simulink model "IFCC_SIMULATION"  (R2018a)
settings: Solver=VariableStepAuto  StartTime=0.0  StopTime=10.0  RelTol=1e-3
libraries: simulink x25
(part 1 of 2)
settings Model: Creator=vsbdh  LastModifiedBy=vsbdh

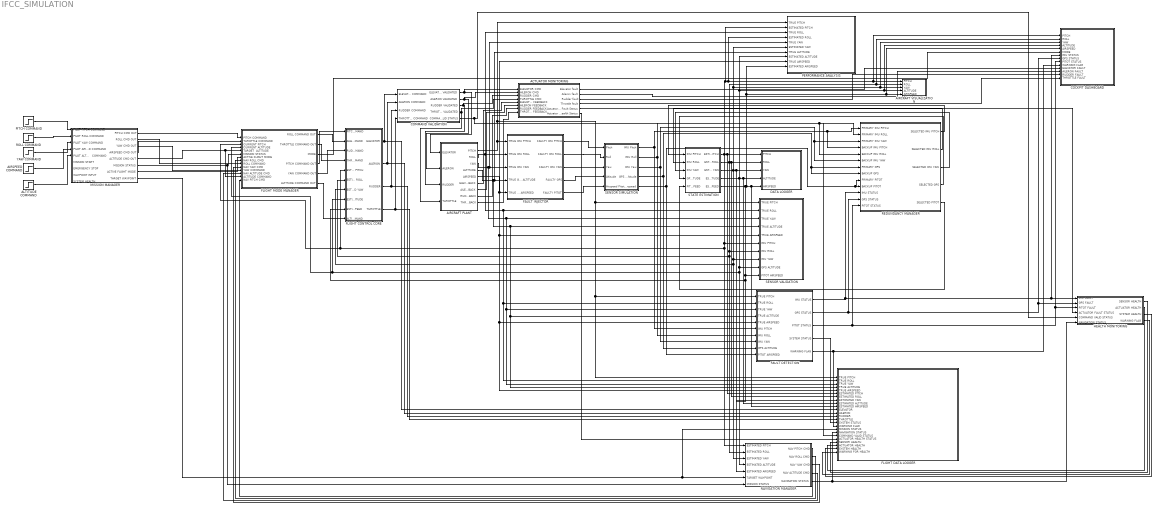
== system IFCC_SIMULATION ==
  " MISSION MANAGER" : Subsystem
  " SENSOR VALIDATION" : Subsystem
  ACTUATOR MONITORING : Subsystem
  AIRCRAFT PLANT : Subsystem
  AIRCRAFT VISUALIZATION : Subsystem
  AIRSPEED COMMAND : Step  Time=0  SampleTime=0
  ALTITUDE COMMAND : Step  Time=2  After=1000  SampleTime=0
  COCKPIT DASHBOARD : Subsystem
  COMMAND VALIDATION : Subsystem
  DATA LOGGER : Subsystem
  FAULT DETECTION : Subsystem
  "FAULT INJECTOR " : Subsystem
  FLIGHT CONTROL CORE : Subsystem
  FLIGHT DATA LOGGER : Subsystem
  FLIGHT MODE MANAGER : Subsystem
  HEALTH MONITORING : Subsystem
  NAVIGATION MANAGER : Subsystem
  PERFORMANCE ANALYSIS : Subsystem
  PITCH COMMAND : Step  Time=0  SampleTime=0
  REDUNDANCY MANAGER : Subsystem
  ROLL COMMAND : Step  Time=0  SampleTime=0
  SENSOR SIMULATION : Subsystem
  STATE ESTIMATION : Subsystem
  YAW COMMAND : Step  Time=0  SampleTime=0
  wires:
  SENSOR SIMULATION/2(IMU Roll) -> REDUNDANCY MANAGER/2(PRIMARY IMU ROLL), REDUNDANCY MANAGER/5(BACKUP IMU ROLL), FAULT DETECTION/7(IMU ROLL)
  FLIGHT CONTROL CORE/4(THROTTLE) -> COMMAND VALIDATION/4(THROTTLE COMMAND), FLIGHT DATA LOGGER/14(THROTTLE)
  REDUNDANCY MANAGER/2(SELECTED IMU ROLL) -> STATE ESTIMATION/2(IMU ROLL)
  "FAULT INJECTOR "/5(FAULTY PITOT) -> SENSOR SIMULATION/5(Airspeed)
  FLIGHT MODE MANAGER/3(MODE) -> COCKPIT DASHBOARD/6(MODE)
  FLIGHT CONTROL CORE/3(RUDDER) -> FLIGHT DATA LOGGER/13(RUDDER), COMMAND VALIDATION/3(RUDDER COMMAND)
  FAULT DETECTION/1(IMU STATUS) -> HEALTH MONITORING/1(IMU FAULT), COCKPIT DASHBOARD/7(IMU STATUS), REDUNDANCY MANAGER/11(IMU STATUS)
  ALTITUDE COMMAND/1 -> " MISSION MANAGER"/5(PILOT ALTITUDE   COMMAND)
  "FAULT INJECTOR "/2(FAULTY IMU ROLL) -> SENSOR SIMULATION/2(Roll)
  "FAULT INJECTOR "/1(FAULTY IMU PITCH) -> SENSOR SIMULATION/1(Pitch)
  "FAULT INJECTOR "/3(FAULTY IMU YAW) -> SENSOR SIMULATION/3(Yaw)
  FAULT DETECTION/5(WARNING FLAG) -> FLIGHT DATA LOGGER/16(WARNING FLAG), COCKPIT DASHBOARD/10(WARNING FLAG)
  REDUNDANCY MANAGER/5(SELECTED PITOT) -> STATE ESTIMATION/5(PITOT AIRSPEED)
  REDUNDANCY MANAGER/3(SELECTED IMU YAW) -> STATE ESTIMATION/3(IMU YAW)
  REDUNDANCY MANAGER/1(SELECTED IMU PITCH) -> STATE ESTIMATION/1(IMU PITCH)
  REDUNDANCY MANAGER/4(SELECTED GPS) -> STATE ESTIMATION/4(GPS ALTITUDE)
  FAULT DETECTION/2(GPS STATUS) -> HEALTH MONITORING/2(GPS FAULT), COCKPIT DASHBOARD/8(GPS STATUS), REDUNDANCY MANAGER/12(GPS STATUS)
  FAULT DETECTION/3(PITOT STATUS) -> HEALTH MONITORING/3(PITOT FAULT), COCKPIT DASHBOARD/9(PITOT STATUS), REDUNDANCY MANAGER/13(PITOT STATUS)
  FAULT DETECTION/4(SYSTEM STATUS) -> FLIGHT DATA LOGGER/15(SYSTEM STATUS)
  YAW COMMAND/1 -> " MISSION MANAGER"/3(PILOT YAW COMMAND)
  FLIGHT MODE MANAGER/1(ROLL COMMAND OUT) -> FLIGHT CONTROL CORE/2(AILERON COMMAND)
  PITCH COMMAND/1 -> " MISSION MANAGER"/1(PILOT PITCH COMMAND)
  FLIGHT CONTROL CORE/1(ELEVATOR) -> COMMAND VALIDATION/1(ELEVATOR COMMAND), FLIGHT DATA LOGGER/11(ELEVATOR)
  FLIGHT MODE MANAGER/2(THROTTLE COMMAND OUT) -> FLIGHT CONTROL CORE/4(THROTTLE COMMAND)
  ROLL COMMAND/1 -> " MISSION MANAGER"/2(PILOT ROLL COMMAND)
  SENSOR SIMULATION/4(GPS Altitude) -> FAULT DETECTION/9(GPS ALTITUDE), REDUNDANCY MANAGER/8(BACKUP GPS), REDUNDANCY MANAGER/7(PRIMARY GPS)
  STATE ESTIMATION/2(ESTIMATED ROLL) -> NAVIGATION MANAGER/2(ESTIMATED ROLL), FLIGHT CONTROL CORE/6(ESTIMATED ROLL), " SENSOR VALIDATION"/7(IMU ROLL), COCKPIT DASHBOARD/2(ROLL), AIRCRAFT VISUALIZATION/2(ROLL), FLIGHT DATA LOGGER/7(ESTIMATED ROLL), DATA LOGGER/2(ROLL)
  AIRSPEED COMMAND/1 -> " MISSION MANAGER"/4(PILOT AIRSPEED COMMAND)
  STATE ESTIMATION/3(ESTIMATED YAW) -> NAVIGATION MANAGER/3(ESTIMATED YAW), FLIGHT CONTROL CORE/7(ESTIMATED YAW), " SENSOR VALIDATION"/8(IMU YAW), PERFORMANCE ANALYSIS/6(ESTIMATED YAW), COCKPIT DASHBOARD/3(YAW), AIRCRAFT VISUALIZATION/3(YAW), FLIGHT DATA LOGGER/8(ESTIMATED YAW), DATA LOGGER/3(YAW)
  STATE ESTIMATION/5(ESTIMATED AIRSPEED) -> PERFORMANCE ANALYSIS/10(ESTIMATED AIRSPEED), COCKPIT DASHBOARD/5(AIRSPEED), AIRCRAFT VISUALIZATION/5(AIRSPEED), FLIGHT DATA LOGGER/10(ESTIMATED AIRSPEED), DATA LOGGER/5(AIRSPEED), NAVIGATION MANAGER/5(ESTIMATED AIRSPEED), FLIGHT CONTROL CORE/9(ESTIMATED AIRSPEED), " SENSOR VALIDATION"/10(PITOT AIRSPEED)
  STATE ESTIMATION/1(ESTIMATED PITCH) -> PERFORMANCE ANALYSIS/2(ESTIMATED PITCH), PERFORMANCE ANALYSIS/4(ESTIMATED ROLL), COCKPIT DASHBOARD/1(PITCH), AIRCRAFT VISUALIZATION/1(PITCH), DATA LOGGER/1(PITCH), FLIGHT DATA LOGGER/6(ESTIMATED PITCH), NAVIGATION MANAGER/1(ESTIMATED PITCH), FLIGHT MODE MANAGER/3(CURRENT PITCH), FLIGHT CONTROL CORE/5(ESTIMATED PITCH), " SENSOR VALIDATION"/6(IMU PITCH)
  FLIGHT CONTROL CORE/2(AILERON) -> COMMAND VALIDATION/2(AILERON COMMAND), FLIGHT DATA LOGGER/12(AILERON)
  SENSOR SIMULATION/5(Pitot Airspeed) -> FAULT DETECTION/10(PITOT AIRSPEED), REDUNDANCY MANAGER/9(PRIMARY PITOT), REDUNDANCY MANAGER/10(BACKUP PITOT)
  AIRCRAFT PLANT/4(ALTITUDE) -> FAULT DETECTION/4(TRUE ALTITUDE), FLIGHT DATA LOGGER/4(TRUE ALTITUDE), " SENSOR VALIDATION"/4(TRUE ALTITUDE), PERFORMANCE ANALYSIS/7(TRUE ALTITUDE), "FAULT INJECTOR "/4(TRUE GPS ALTITUDE)
  SENSOR SIMULATION/3(IMU Yaw) -> FAULT DETECTION/8(IMU YAW), REDUNDANCY MANAGER/3(PRIMARY IMU YAW), REDUNDANCY MANAGER/6(BACKUP IMU YAW)
  AIRCRAFT PLANT/3(YAW) -> FLIGHT DATA LOGGER/3(TRUE YAW), FAULT DETECTION/3(TRUE YAW), " SENSOR VALIDATION"/3(TRUE YAW), PERFORMANCE ANALYSIS/5(TRUE YAW), "FAULT INJECTOR "/3(TRUE IMU YAW)
  AIRCRAFT PLANT/2(ROLL) -> " SENSOR VALIDATION"/2(TRUE ROLL), FAULT DETECTION/2(TRUE ROLL), FLIGHT DATA LOGGER/2(TRUE ROLL), PERFORMANCE ANALYSIS/3(TRUE ROLL), "FAULT INJECTOR "/2(TRUE IMU ROLL)
  STATE ESTIMATION/4(ESTIMATED ALTITUDE) -> PERFORMANCE ANALYSIS/8(ESTIMATED ALTITUDE), COCKPIT DASHBOARD/4(ALTITUDE), AIRCRAFT VISUALIZATION/4(ALTITUDE), FLIGHT DATA LOGGER/9(ESTIMATED ALTITUDE), DATA LOGGER/4(ALTITUDE), NAVIGATION MANAGER/4(ESTIMATED ALTITUDE), FLIGHT CONTROL CORE/8(ESTIMATED ALTITUDE), FLIGHT MODE MANAGER/4(CURRENT ALTITUDE), " SENSOR VALIDATION"/9(GPS ALTITUDE)
  SENSOR SIMULATION/1(IMU Pitch) -> FAULT DETECTION/6(IMU PITCH), REDUNDANCY MANAGER/1(PRIMARY IMU PITCH), REDUNDANCY MANAGER/4(BACKUP IMU PITCH)
  AIRCRAFT PLANT/5(AIRSPEED) -> " SENSOR VALIDATION"/5(TRUE AIRSPEED), FAULT DETECTION/5(TRUE AIRSPEED), FLIGHT DATA LOGGER/5(TRUE AIRSPEED), PERFORMANCE ANALYSIS/9(TRUE AIRSPEED), "FAULT INJECTOR "/5(TRUE PITOT AIRSPEED)
  AIRCRAFT PLANT/1(PITCH) -> "FAULT INJECTOR "/1(TRUE IMU PITCH), PERFORMANCE ANALYSIS/1(TRUE PITCH), FLIGHT DATA LOGGER/1(TRUE PITCH), FAULT DETECTION/1(TRUE PITCH), " SENSOR VALIDATION"/1(TRUE PITCH)
  "FAULT INJECTOR "/4(FAULTY GPS) -> SENSOR SIMULATION/4(Altitude)
  " MISSION MANAGER"/1(" PITCH CMD OUT") -> FLIGHT MODE MANAGER/1(PITCH COMMAND)
  " MISSION MANAGER"/4(AIRSPEED CMD OUT) -> FLIGHT MODE MANAGER/2(THROTTLE COMMAND)
  COMMAND VALIDATION/1(ELEVATOR VALIDATED) -> ACTUATOR MONITORING/1(ELEVATOR CMD), AIRCRAFT PLANT/1(ELEVATOR)
  COMMAND VALIDATION/2(AILERON VALIDATED) -> ACTUATOR MONITORING/2(AILERON CMD), AIRCRAFT PLANT/2(AILERON)
  COMMAND VALIDATION/3(RUDDER VALIDATED) -> ACTUATOR MONITORING/3(RUDDER CMD), AIRCRAFT PLANT/3(RUDDER)
  COMMAND VALIDATION/4(THROTTLE VALIDATED) -> ACTUATOR MONITORING/4(THROTTLE CMD), AIRCRAFT PLANT/4(THROTTLE)
  AIRCRAFT PLANT/6(ELEVATOR FEEDBACK) -> ACTUATOR MONITORING/5(ELEVATOR FEEDBACK)
  AIRCRAFT PLANT/7(AILERON FEEDBACK) -> ACTUATOR MONITORING/6(AILERON FEEDBACK)
  AIRCRAFT PLANT/8(RUDDER FEEDBACK) -> ACTUATOR MONITORING/7(RUDDER FEEDBACK)
  AIRCRAFT PLANT/9(THROTTLE FEEDBACK) -> ACTUATOR MONITORING/8(THROTTLE FEEDBACK)
  " MISSION MANAGER"/6(MISSION STATUS) -> NAVIGATION MANAGER/7(MISSION STATUS), FLIGHT MODE MANAGER/6(MISSION STATUS)
  " MISSION MANAGER"/8(TARGET WAYPOINT) -> FLIGHT DATA LOGGER/17(MISSION STATUS), NAVIGATION MANAGER/6(TARGET WAYPOINT)
  ACTUATOR MONITORING/5(Actuator Fault Status) -> HEALTH MONITORING/4(ACTUATOR FAULT STATUS)
  NAVIGATION MANAGER/5(NAVIGATION STATUS) -> FLIGHT DATA LOGGER/18(NAVIGATION STATUS), HEALTH MONITORING/6(NAVIGATION STATUS)
  COMMAND VALIDATION/5(COMMAND VALID STATUS) -> FLIGHT DATA LOGGER/19(COMMAND VALID STATUS), HEALTH MONITORING/5(COMMAND VALID STATUS)
  ACTUATOR MONITORING/6(Actuator Health Status) -> FLIGHT DATA LOGGER/20(ACTUATOR HEALTH STATUS)
  HEALTH MONITORING/1(SENSOR HEALTH) -> FLIGHT DATA LOGGER/21(SENSOR HEALTH)
  HEALTH MONITORING/2(ACTUATOR HEALTH) -> FLIGHT DATA LOGGER/22(ACTUATOR HEALTH)
  HEALTH MONITORING/3(SYSTEM HEALTH) -> FLIGHT DATA LOGGER/23(SYSTEM HEALTH)
  HEALTH MONITORING/4(WARNING FLAG) -> FLIGHT DATA LOGGER/24(WARNING FOR HEALTH)
  ACTUATOR MONITORING/1(Elevator fault) -> COCKPIT DASHBOARD/11(ELEVATOR FAULT)
  ACTUATOR MONITORING/2(Aileron fault) -> COCKPIT DASHBOARD/12(AILERON FAULT)
  ACTUATOR MONITORING/4(Throttle fault) -> COCKPIT DASHBOARD/14(THROTTLE FAULT)
  ACTUATOR MONITORING/3(Rudder fault) -> COCKPIT DASHBOARD/13(RUDDER FAULT)
  " MISSION MANAGER"/7(ACTIVE FLIGHT MODE) -> FLIGHT MODE MANAGER/7(ACTIVE FLIGHT MODE)
  FLIGHT MODE MANAGER/4("PITCH COMMAND OUT ") -> FLIGHT CONTROL CORE/1(PITCH COMMAND)
  FLIGHT MODE MANAGER/5(YAW COMMAND OUT) -> FLIGHT CONTROL CORE/3(RUDDER COMMAND)
  FLIGHT MODE MANAGER/6(ALTITUDE COMMAND OUT) -> FLIGHT CONTROL CORE/10(ALTITUDE COMMAND)
  " MISSION MANAGER"/2(ROLL CMD OUT) -> FLIGHT MODE MANAGER/9(ROLL COMMAND)
  " MISSION MANAGER"/3(YAW CMD OUT) -> FLIGHT MODE MANAGER/11(YAW COMMAND)
  " MISSION MANAGER"/5(ALTITUDE CMD OUT) -> FLIGHT MODE MANAGER/13(ALTITUDE COMMAND), FLIGHT MODE MANAGER/5(TARGET  ALTITUDE)
  NAVIGATION MANAGER/2(NAV ROLL CMD) -> FLIGHT MODE MANAGER/8(NAV ROLL CMD)
  NAVIGATION MANAGER/1(NAV PITCH CMD) -> FLIGHT MODE MANAGER/14(NAV PITCH CMD)
  NAVIGATION MANAGER/3(NAV YAW CMD) -> FLIGHT MODE MANAGER/10(NAV YAW CMD)
  NAVIGATION MANAGER/4(NAV ALTITUDE CMD) -> FLIGHT MODE MANAGER/12(NAV ALTITUDE CMD)

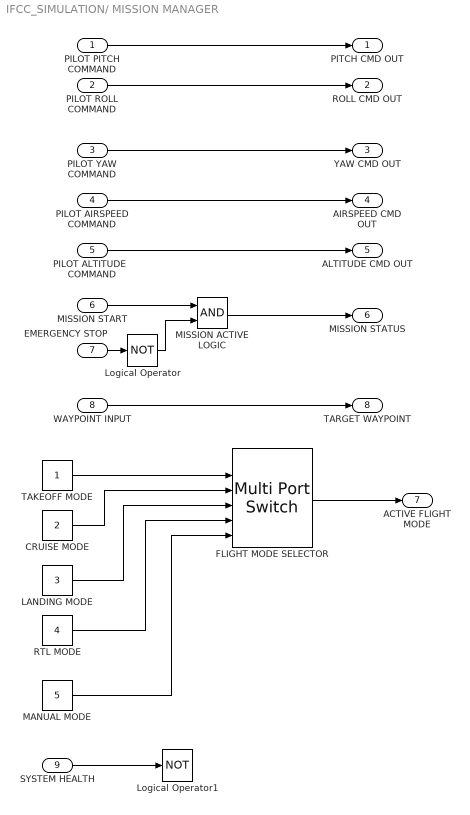
== system IFCC_SIMULATION/ MISSION MANAGER ==
  PILOT PITCH COMMAND : Inport
  PILOT ROLL COMMAND : Inport  Port=2
  PILOT YAW COMMAND : Inport  Port=3
  PILOT AIRSPEED COMMAND : Inport  Port=4
  PILOT ALTITUDE   COMMAND : Inport  Port=5
  MISSION START : Inport  Port=6
  EMERGENCY STOP : Inport  Port=7
  WAYPOINT INPUT : Inport  Port=8
  "SYSTEM HEALTH " : Inport  Port=9
  CRUISE MODE : Constant  Value=2
  FLIGHT MODE SELECTOR : MultiPortSwitch  Inputs=5
  LANDING MODE : Constant  Value=3
  Logical Operator : Logic  Operator=NOT  AllPortsSameDT=off  OutDataTypeStr=boolean
  Logical Operator1 : Logic  Operator=NOT  AllPortsSameDT=off  OutDataTypeStr=boolean
  MANUAL MODE : Constant  Value=5
  MISSION ACTIVE LOGIC : Logic  AllPortsSameDT=off  OutDataTypeStr=boolean
  RTL MODE : Constant  Value=4
  TAKEOFF MODE : Constant
  " PITCH CMD OUT" : Outport
  ROLL CMD OUT : Outport  Port=2
  YAW CMD OUT : Outport  Port=3
  AIRSPEED CMD OUT : Outport  Port=4
  ALTITUDE CMD OUT : Outport  Port=5
  MISSION STATUS : Outport  Port=6
  ACTIVE FLIGHT MODE : Outport  Port=7
  TARGET WAYPOINT : Outport  Port=8
  wires:
  MISSION START/1 -> MISSION ACTIVE LOGIC/1
  MISSION ACTIVE LOGIC/1 -> MISSION STATUS/1
  PILOT PITCH COMMAND/1 -> " PITCH CMD OUT"/1
  PILOT ROLL COMMAND/1 -> ROLL CMD OUT/1
  PILOT YAW COMMAND/1 -> YAW CMD OUT/1
  TAKEOFF MODE/1 -> FLIGHT MODE SELECTOR/2
  CRUISE MODE/1 -> FLIGHT MODE SELECTOR/3
  LANDING MODE/1 -> FLIGHT MODE SELECTOR/4
  RTL MODE/1 -> FLIGHT MODE SELECTOR/5
  MANUAL MODE/1 -> FLIGHT MODE SELECTOR/6
  FLIGHT MODE SELECTOR/1 -> ACTIVE FLIGHT MODE/1
  PILOT AIRSPEED COMMAND/1 -> AIRSPEED CMD OUT/1
  PILOT ALTITUDE   COMMAND/1 -> ALTITUDE CMD OUT/1
  WAYPOINT INPUT/1 -> TARGET WAYPOINT/1
  EMERGENCY STOP/1 -> Logical Operator/1
  Logical Operator/1 -> MISSION ACTIVE LOGIC/2
  "SYSTEM HEALTH "/1 -> Logical Operator1/1

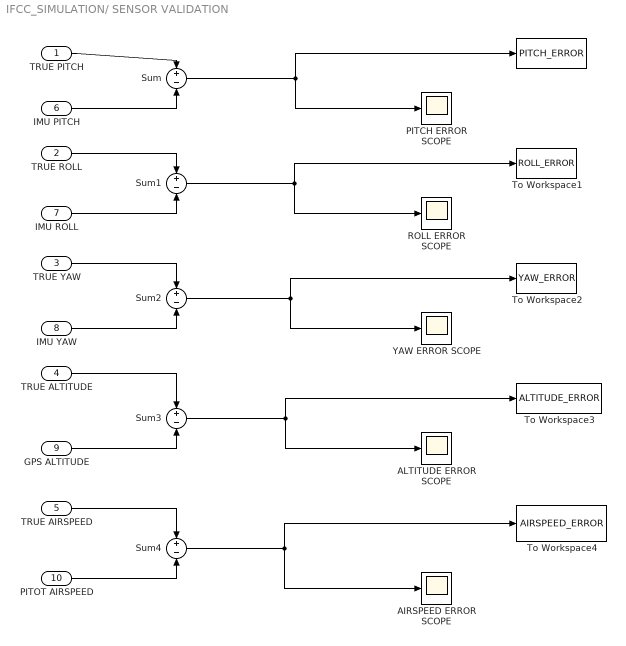
== system IFCC_SIMULATION/ SENSOR VALIDATION ==
  TRUE PITCH : Inport
  TRUE ROLL : Inport  Port=2
  TRUE YAW : Inport  Port=3
  TRUE ALTITUDE : Inport  Port=4
  TRUE AIRSPEED : Inport  Port=5
  IMU PITCH : Inport  Port=6
  IMU ROLL : Inport  Port=7
  IMU YAW : Inport  Port=8
  GPS ALTITUDE : Inport  Port=9
  PITOT AIRSPEED : Inport  Port=10
  " " : ToWorkspace  VariableName=PITCH_ERROR  SaveFormat=Structure With Time  SampleTime=-1
  AIRSPEED ERROR SCOPE : Scope
  ALTITUDE ERROR SCOPE : Scope
  PITCH ERROR SCOPE : Scope
  ROLL ERROR SCOPE : Scope
  Sum{,1..4} (5 alike) : Sum  Inputs=+-
  To Workspace1 : ToWorkspace  VariableName=ROLL_ERROR  SaveFormat=Structure With Time  SampleTime=-1
  To Workspace2 : ToWorkspace  VariableName=YAW_ERROR  SaveFormat=Structure With Time  SampleTime=-1
  To Workspace3 : ToWorkspace  VariableName=ALTITUDE_ERROR  SaveFormat=Structure With Time  SampleTime=-1
  To Workspace4 : ToWorkspace  VariableName=AIRSPEED_ERROR  SaveFormat=Structure With Time  SampleTime=-1
  YAW ERROR SCOPE : Scope
  wires:
  TRUE PITCH/1 -> Sum/1
  IMU PITCH/1 -> Sum/2
  Sum/1 -> " "/1, PITCH ERROR SCOPE/1
  TRUE ROLL/1 -> Sum1/1
  IMU ROLL/1 -> Sum1/2
  Sum1/1 -> To Workspace1/1, ROLL ERROR SCOPE/1
  TRUE YAW/1 -> Sum2/1
  IMU YAW/1 -> Sum2/2
  Sum2/1 -> To Workspace2/1, YAW ERROR SCOPE/1
  TRUE ALTITUDE/1 -> Sum3/1
  GPS ALTITUDE/1 -> Sum3/2
  Sum3/1 -> To Workspace3/1, ALTITUDE ERROR SCOPE/1
  TRUE AIRSPEED/1 -> Sum4/1
  PITOT AIRSPEED/1 -> Sum4/2
  Sum4/1 -> AIRSPEED ERROR SCOPE/1, To Workspace4/1

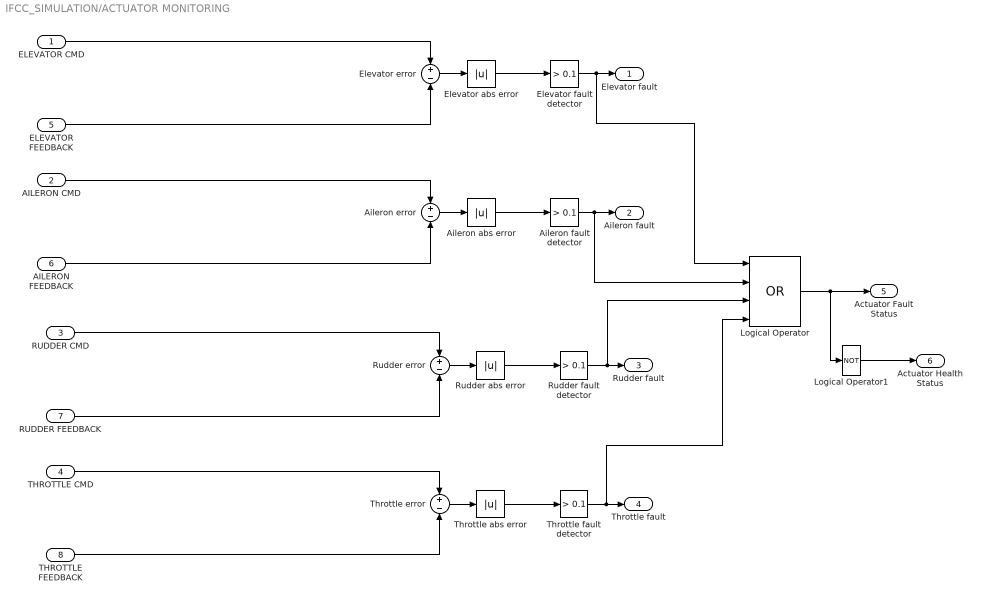
== system IFCC_SIMULATION/ACTUATOR MONITORING ==
  ELEVATOR CMD : Inport
  AILERON CMD : Inport  Port=2
  RUDDER CMD : Inport  Port=3
  THROTTLE CMD : Inport  Port=4
  ELEVATOR FEEDBACK : Inport  Port=5
  AILERON FEEDBACK : Inport  Port=6
  RUDDER FEEDBACK : Inport  Port=7
  THROTTLE FEEDBACK : Inport  Port=8
  " Aileron error" : Sum  Inputs=+-
  " Elevator error" : Sum  Inputs=+-
  " Rudder error" : Sum  Inputs=+-
  " Throttle error" : Sum  Inputs=+-
  Aileron abs error : Abs
  Aileron fault detector : simulink/Logic and Bit Operations/Compare To Constant  relop=>  const=0.1  OutDataTypeStr=boolean
  Elevator abs error : Abs
  Elevator fault detector : simulink/Logic and Bit Operations/Compare To Constant  relop=>  const=0.1  OutDataTypeStr=boolean
  Logical Operator : Logic  Operator=OR  Inputs=4  AllPortsSameDT=off  OutDataTypeStr=boolean
  Logical Operator1 : Logic  Operator=NOT  Inputs=4  AllPortsSameDT=off  OutDataTypeStr=boolean
  Rudder abs error : Abs
  Rudder fault detector : simulink/Logic and Bit Operations/Compare To Constant  relop=>  const=0.1  OutDataTypeStr=boolean
  Throttle abs error : Abs
  Throttle fault detector : simulink/Logic and Bit Operations/Compare To Constant  relop=>  const=0.1  OutDataTypeStr=boolean
  Elevator fault : Outport
  Aileron fault : Outport  Port=2
  Rudder fault : Outport  Port=3
  Throttle fault : Outport  Port=4
  Actuator Fault Status : Outport  Port=5
  Actuator Health Status : Outport  Port=6
  wires:
  ELEVATOR CMD/1 -> " Elevator error"/1
  ELEVATOR FEEDBACK/1 -> " Elevator error"/2
  " Elevator error"/1 -> Elevator abs error/1
  Elevator abs error/1 -> Elevator fault detector/1
  Elevator fault detector/1 -> Logical Operator/1, Elevator fault/1
  Aileron fault detector/1 -> Logical Operator/2, Aileron fault/1
  Aileron abs error/1 -> Aileron fault detector/1
  " Aileron error"/1 -> Aileron abs error/1
  AILERON CMD/1 -> " Aileron error"/1
  AILERON FEEDBACK/1 -> " Aileron error"/2
  Rudder fault detector/1 -> Logical Operator/3, Rudder fault/1
  Rudder abs error/1 -> Rudder fault detector/1
  " Rudder error"/1 -> Rudder abs error/1
  RUDDER CMD/1 -> " Rudder error"/1
  RUDDER FEEDBACK/1 -> " Rudder error"/2
  Throttle fault detector/1 -> Logical Operator/4, Throttle fault/1
  Throttle abs error/1 -> Throttle fault detector/1
  " Throttle error"/1 -> Throttle abs error/1
  THROTTLE CMD/1 -> " Throttle error"/1
  THROTTLE FEEDBACK/1 -> " Throttle error"/2
  Logical Operator/1 -> Logical Operator1/1, Actuator Fault Status/1
  Logical Operator1/1 -> Actuator Health Status/1

== system IFCC_SIMULATION/AIRCRAFT PLANT ==
  ELEVATOR : Inport
  AILERON : Inport  Port=2
  RUDDER : Inport  Port=3
  THROTTLE : Inport  Port=4
  AILERON ACTUATOR : TransferFcn  Denominator=[0.1 1]
  AIRSPEED DYNAMICS : Subsystem
  ALTITUDE DYNAMICS : Subsystem
  ELEVATOR ACTUATOR : TransferFcn  Denominator=[0.1 1]
  PITCH DYNAMICS : Subsystem
  ROLL DYNAMICS : Subsystem
  RUDDER  ACTUATOR : TransferFcn  Denominator=[0.1 1]
  THROTTLE  ACTUATOR : TransferFcn  Denominator=[0.2 1]
  YAW DYNAMICS : Subsystem
  PITCH : Outport
  ROLL : Outport  Port=2
  YAW : Outport  Port=3
  ALTITUDE : Outport  Port=4
  AIRSPEED : Outport  Port=5
  ELEVATOR FEEDBACK : Outport  Port=6
  AILERON FEEDBACK : Outport  Port=7
  RUDDER FEEDBACK : Outport  Port=8
  THROTTLE FEEDBACK : Outport  Port=9
  wires:
  PITCH DYNAMICS/1(PITCH) -> PITCH/1, ALTITUDE DYNAMICS/1(PITCH)
  ALTITUDE DYNAMICS/1(ALTITUDE) -> ALTITUDE/1
  ROLL DYNAMICS/1(ROLL) -> ROLL/1
  YAW DYNAMICS/1(YAW) -> YAW/1
  AIRSPEED DYNAMICS/1(AIRSPEED) -> AIRSPEED/1
  ELEVATOR/1 -> ELEVATOR ACTUATOR/1
  ELEVATOR ACTUATOR/1 -> ELEVATOR FEEDBACK/1, PITCH DYNAMICS/1(ELEVATOR)
  AILERON ACTUATOR/1 -> AILERON FEEDBACK/1, ROLL DYNAMICS/1(AILERON)
  AILERON/1 -> AILERON ACTUATOR/1
  RUDDER  ACTUATOR/1 -> RUDDER FEEDBACK/1, YAW DYNAMICS/1(RUDDER)
  RUDDER/1 -> RUDDER  ACTUATOR/1
  THROTTLE/1 -> THROTTLE  ACTUATOR/1
  THROTTLE  ACTUATOR/1 -> THROTTLE FEEDBACK/1, AIRSPEED DYNAMICS/1("THROTTLE ")

== system IFCC_SIMULATION/AIRCRAFT VISUALIZATION ==
  PITCH : Inport
  ROLL : Inport  Port=2
  YAW : Inport  Port=3
  ALTITUDE : Inport  Port=4
  AIRSPEED : Inport  Port=5
  AIRSPEED SCOPE : Scope
  ALTITUDE SCOPE : Scope
  PITCH SCOPE : Scope
  ROLL SCOPE : Scope
  YAW SCOPE : Scope
  wires:
  PITCH/1 -> PITCH SCOPE/1
  ROLL/1 -> ROLL SCOPE/1
  YAW/1 -> YAW SCOPE/1
  ALTITUDE/1 -> ALTITUDE SCOPE/1
  AIRSPEED/1 -> AIRSPEED SCOPE/1

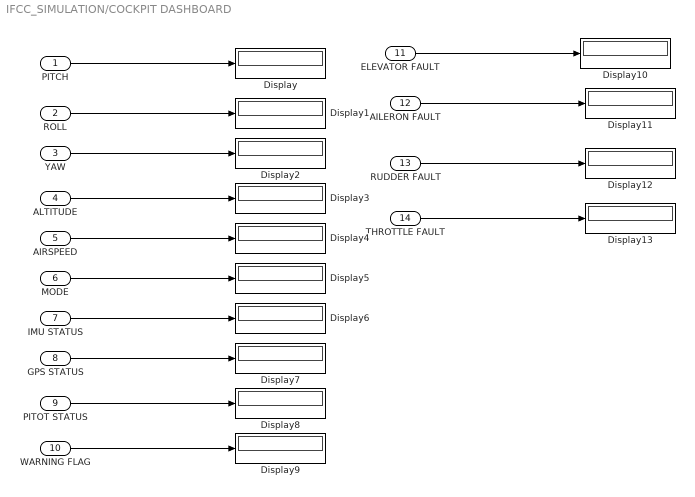
== system IFCC_SIMULATION/COCKPIT DASHBOARD ==
  PITCH : Inport
  ROLL : Inport  Port=2
  YAW : Inport  Port=3
  ALTITUDE : Inport  Port=4
  AIRSPEED : Inport  Port=5
  MODE : Inport  Port=6
  IMU STATUS : Inport  Port=7
  GPS STATUS : Inport  Port=8
  PITOT STATUS : Inport  Port=9
  WARNING FLAG : Inport  Port=10
  ELEVATOR FAULT : Inport  Port=11
  AILERON FAULT : Inport  Port=12
  RUDDER FAULT : Inport  Port=13
  THROTTLE FAULT : Inport  Port=14
  Display{,1..13} (14 alike) : Display
  wires:
  PITCH/1 -> Display/1
  ROLL/1 -> Display1/1
  YAW/1 -> Display2/1
  ALTITUDE/1 -> Display3/1
  AIRSPEED/1 -> Display4/1
  MODE/1 -> Display5/1
  IMU STATUS/1 -> Display6/1
  GPS STATUS/1 -> Display7/1
  PITOT STATUS/1 -> Display8/1
  WARNING FLAG/1 -> Display9/1
  ELEVATOR FAULT/1 -> Display10/1
  AILERON FAULT/1 -> Display11/1
  RUDDER FAULT/1 -> Display12/1
  THROTTLE FAULT/1 -> Display13/1

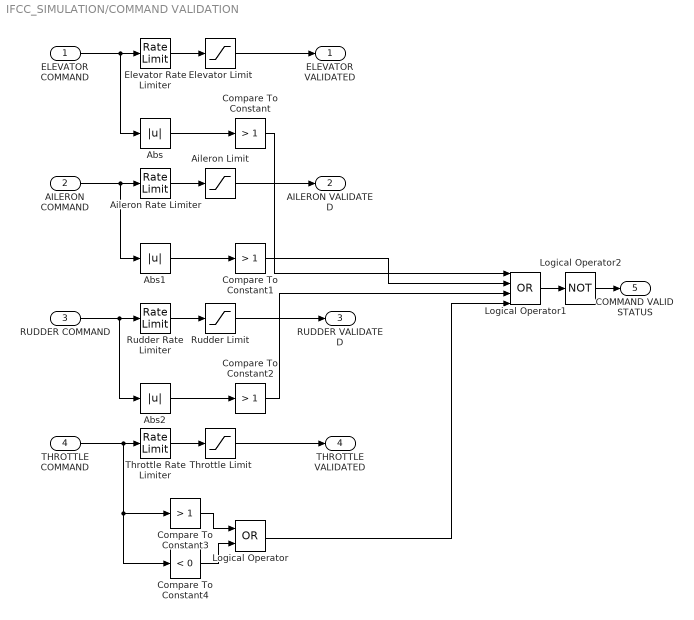
== system IFCC_SIMULATION/COMMAND VALIDATION ==
  ELEVATOR COMMAND : Inport
  AILERON COMMAND : Inport  Port=2
  RUDDER COMMAND : Inport  Port=3
  THROTTLE COMMAND : Inport  Port=4
  Abs : Abs
  Abs1 : Abs
  Abs2 : Abs
  Aileron Rate Limiter : RateLimiter  RisingSlewLimit=2  FallingSlewLimit=-2  SampleTimeMode=inherited
  Aileron Limit : Saturate  UpperLimit=1  LowerLimit=-1
  Compare To Constant{,1..3} (4 alike) : simulink/Logic and Bit Operations/Compare To Constant  relop=>  const=1  OutDataTypeStr=boolean
  Compare To Constant4 : simulink/Logic and Bit Operations/Compare To Constant  relop=<  const=0  OutDataTypeStr=boolean
  Elevator Rate Limiter : RateLimiter  RisingSlewLimit=2  FallingSlewLimit=-2  SampleTimeMode=inherited
  Elevator Limit : Saturate  UpperLimit=1  LowerLimit=-1
  Logical Operator : Logic  Operator=OR  AllPortsSameDT=off  OutDataTypeStr=boolean
  Logical Operator1 : Logic  Operator=OR  Inputs=4  AllPortsSameDT=off  OutDataTypeStr=boolean
  Logical Operator2 : Logic  Operator=NOT  Inputs=4  AllPortsSameDT=off  OutDataTypeStr=boolean
  Rudder Rate Limiter : RateLimiter  RisingSlewLimit=1.5  FallingSlewLimit=-1.5  SampleTimeMode=inherited
  Rudder Limit : Saturate  UpperLimit=1  LowerLimit=-1
  Throttle Rate Limiter : RateLimiter  RisingSlewLimit=0.5  FallingSlewLimit=-0.5  SampleTimeMode=inherited
  Throttle Limit : Saturate  UpperLimit=1  LowerLimit=0
  ELEVATOR VALIDATED : Outport
  AILERON VALIDATED : Outport  Port=2
  RUDDER VALIDATED : Outport  Port=3
  THROTTLE VALIDATED : Outport  Port=4
  COMMAND VALID STATUS : Outport  Port=5
  wires:
  ELEVATOR COMMAND/1 -> Abs/1, Elevator Rate Limiter/1
  Elevator Rate Limiter/1 -> Elevator Limit/1
  Elevator Limit/1 -> ELEVATOR VALIDATED/1
  Aileron Rate Limiter/1 -> Aileron Limit/1
  Aileron Limit/1 -> AILERON VALIDATED/1
  Rudder Rate Limiter/1 -> Rudder Limit/1
  Rudder Limit/1 -> RUDDER VALIDATED/1
  THROTTLE COMMAND/1 -> Compare To Constant4/1, Compare To Constant3/1, Throttle Rate Limiter/1
  Throttle Rate Limiter/1 -> Throttle Limit/1
  Throttle Limit/1 -> THROTTLE VALIDATED/1
  Abs/1 -> Compare To Constant/1
  Abs1/1 -> Compare To Constant1/1
  AILERON COMMAND/1 -> Abs1/1, Aileron Rate Limiter/1
  Abs2/1 -> Compare To Constant2/1
  RUDDER COMMAND/1 -> Abs2/1, Rudder Rate Limiter/1
  Compare To Constant3/1 -> Logical Operator/1
  Compare To Constant4/1 -> Logical Operator/2
  Compare To Constant1/1 -> Logical Operator1/2
  Compare To Constant2/1 -> Logical Operator1/3
  Compare To Constant/1 -> Logical Operator1/1
  Logical Operator/1 -> Logical Operator1/4
  Logical Operator1/1 -> Logical Operator2/1
  Logical Operator2/1 -> COMMAND VALID STATUS/1

== system IFCC_SIMULATION/DATA LOGGER ==
  PITCH : Inport
  ROLL : Inport  Port=2
  YAW : Inport  Port=3
  ALTITUDE : Inport  Port=4
  AIRSPEED : Inport  Port=5
  AIRSPEED DATA : ToWorkspace  VariableName=airspeed_data  SaveFormat=Structure With Time  SampleTime=-1
  ALTITUDE DATA : ToWorkspace  VariableName=altitude_data  SaveFormat=Structure With Time  SampleTime=-1
  PITCH DATA : ToWorkspace  VariableName=pitch_data  SaveFormat=Structure With Time  SampleTime=-1
  ROLL DATA : ToWorkspace  VariableName=roll_data  SaveFormat=Structure With Time  SampleTime=-1
  YAW DATA : ToWorkspace  VariableName=yaw_data  SaveFormat=Structure With Time  SampleTime=-1
  wires:
  PITCH/1 -> PITCH DATA/1
  ROLL/1 -> ROLL DATA/1
  YAW/1 -> YAW DATA/1
  ALTITUDE/1 -> ALTITUDE DATA/1
  AIRSPEED/1 -> AIRSPEED DATA/1

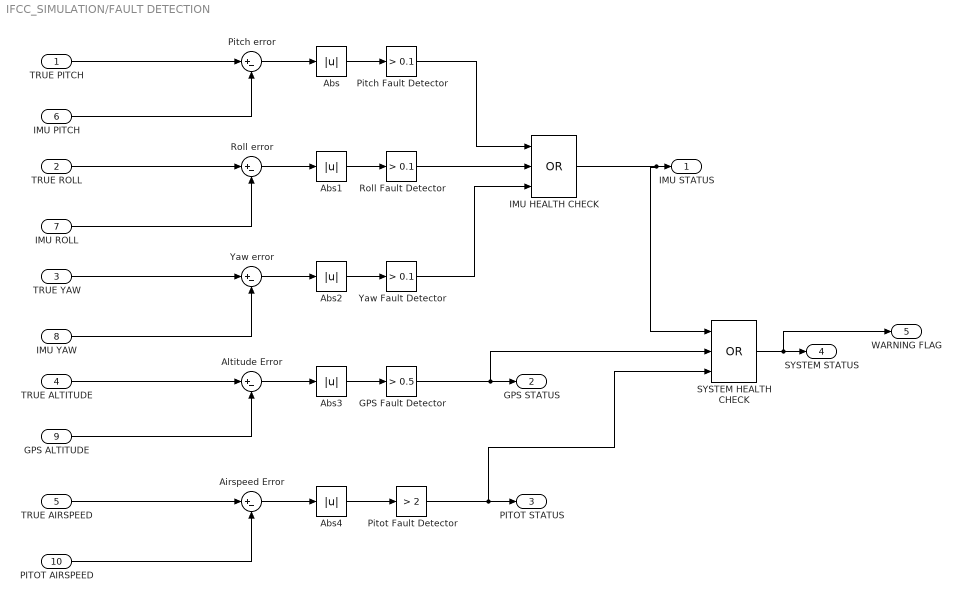
== system IFCC_SIMULATION/FAULT DETECTION ==
  TRUE PITCH : Inport
  TRUE ROLL : Inport  Port=2
  TRUE YAW : Inport  Port=3
  TRUE ALTITUDE : Inport  Port=4
  TRUE AIRSPEED : Inport  Port=5
  IMU PITCH : Inport  Port=6
  IMU ROLL : Inport  Port=7
  IMU YAW : Inport  Port=8
  GPS ALTITUDE : Inport  Port=9
  PITOT AIRSPEED : Inport  Port=10
  " Airspeed Error" : Sum  Inputs=|+-
  " Altitude Error" : Sum  Inputs=|+-
  " Pitch error" : Sum  Inputs=|+-
  " Roll error" : Sum  Inputs=|+-
  " Yaw error" : Sum  Inputs=|+-
  Abs{,1..4} (5 alike) : Abs
  GPS Fault Detector : simulink/Logic and Bit Operations/Compare To Constant  relop=>  const=0.5  OutDataTypeStr=boolean
  IMU HEALTH CHECK : Logic  Operator=OR  Inputs=3  AllPortsSameDT=off  OutDataTypeStr=boolean
  Pitch Fault Detector : simulink/Logic and Bit Operations/Compare To Constant  relop=>  const=0.1  OutDataTypeStr=boolean
  Pitot Fault Detector : simulink/Logic and Bit Operations/Compare To Constant  relop=>  const=2  OutDataTypeStr=boolean
  Roll Fault Detector : simulink/Logic and Bit Operations/Compare To Constant  relop=>  const=0.1  OutDataTypeStr=boolean
  SYSTEM HEALTH CHECK : Logic  Operator=OR  Inputs=3  AllPortsSameDT=off  OutDataTypeStr=boolean
  Yaw Fault Detector : simulink/Logic and Bit Operations/Compare To Constant  relop=>  const=0.1  OutDataTypeStr=boolean
  IMU STATUS : Outport
  GPS STATUS : Outport  Port=2
  PITOT STATUS : Outport  Port=3
  SYSTEM STATUS : Outport  Port=4
  WARNING FLAG : Outport  Port=5
  wires:
  TRUE PITCH/1 -> " Pitch error"/1
  IMU PITCH/1 -> " Pitch error"/2
  TRUE ROLL/1 -> " Roll error"/1
  IMU ROLL/1 -> " Roll error"/2
  " Pitch error"/1 -> Abs/1
  Abs/1 -> Pitch Fault Detector/1
  " Roll error"/1 -> Abs1/1
  Abs1/1 -> Roll Fault Detector/1
  TRUE YAW/1 -> " Yaw error"/1
  IMU YAW/1 -> " Yaw error"/2
  " Yaw error"/1 -> Abs2/1
  Abs2/1 -> Yaw Fault Detector/1
  Roll Fault Detector/1 -> IMU HEALTH CHECK/2
  Pitch Fault Detector/1 -> IMU HEALTH CHECK/1
  Yaw Fault Detector/1 -> IMU HEALTH CHECK/3
  IMU HEALTH CHECK/1 -> SYSTEM HEALTH CHECK/1, IMU STATUS/1
  " Altitude Error"/1 -> Abs3/1
  TRUE ALTITUDE/1 -> " Altitude Error"/1
  GPS ALTITUDE/1 -> " Altitude Error"/2
  Abs3/1 -> GPS Fault Detector/1
  GPS Fault Detector/1 -> SYSTEM HEALTH CHECK/2, GPS STATUS/1
  TRUE AIRSPEED/1 -> " Airspeed Error"/1
  PITOT AIRSPEED/1 -> " Airspeed Error"/2
  " Airspeed Error"/1 -> Abs4/1
  Abs4/1 -> Pitot Fault Detector/1
  Pitot Fault Detector/1 -> SYSTEM HEALTH CHECK/3, PITOT STATUS/1
  SYSTEM HEALTH CHECK/1 -> WARNING FLAG/1, SYSTEM STATUS/1

== system IFCC_SIMULATION/FAULT INJECTOR  ==
  TRUE IMU PITCH : Inport
  TRUE IMU ROLL : Inport  Port=2
  TRUE IMU YAW : Inport  Port=3
  TRUE GPS ALTITUDE : Inport  Port=4
  TRUE PITOT AIRSPEED : Inport  Port=5
  Constant : Constant  Value=10
  Constant1 : Constant  Value=10
  Constant2 : Constant  Value=10
  Constant3 : Constant  Value=500
  Constant4 : Constant  Value=200
  Manual Switch{,1..4} (5 alike) : ManualSwitch
  FAULTY IMU PITCH : Outport
  FAULTY IMU ROLL : Outport  Port=2
  FAULTY IMU YAW : Outport  Port=3
  FAULTY GPS : Outport  Port=4
  FAULTY PITOT : Outport  Port=5
  wires:
  TRUE IMU PITCH/1 -> Manual Switch/1
  Constant/1 -> Manual Switch/2
  Manual Switch/1 -> FAULTY IMU PITCH/1
  TRUE IMU ROLL/1 -> Manual Switch1/1
  Manual Switch1/1 -> FAULTY IMU ROLL/1
  Constant1/1 -> Manual Switch1/2
  TRUE IMU YAW/1 -> Manual Switch2/1
  Manual Switch2/1 -> FAULTY IMU YAW/1
  Constant2/1 -> Manual Switch2/2
  TRUE GPS ALTITUDE/1 -> Manual Switch3/1
  Constant3/1 -> Manual Switch3/2
  Manual Switch3/1 -> FAULTY GPS/1
  TRUE PITOT AIRSPEED/1 -> Manual Switch4/1
  Manual Switch4/1 -> FAULTY PITOT/1
  Constant4/1 -> Manual Switch4/2

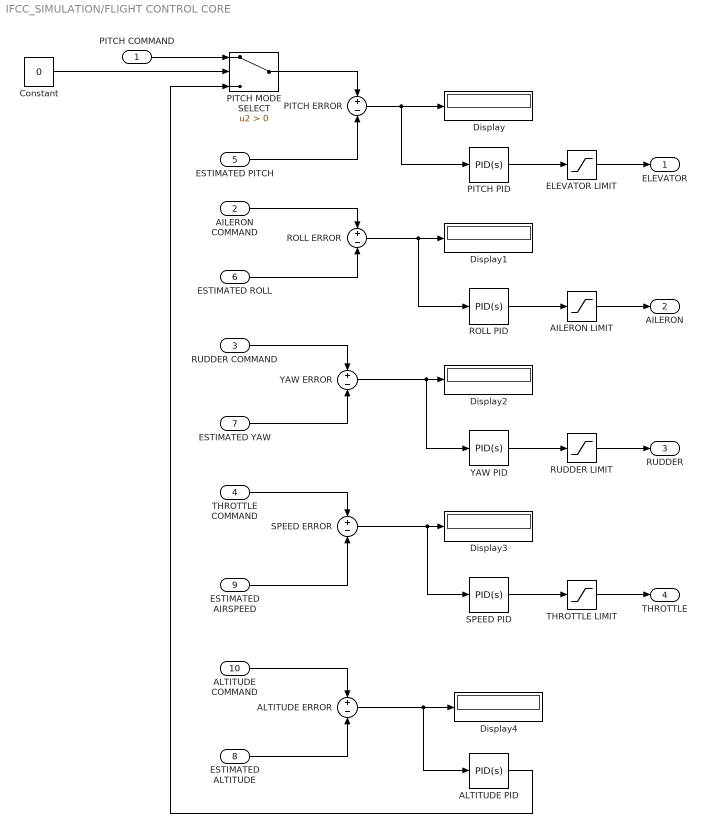
== system IFCC_SIMULATION/FLIGHT CONTROL CORE ==
  PITCH COMMAND : Inport
  AILERON COMMAND : Inport  Port=2
  RUDDER COMMAND : Inport  Port=3
  THROTTLE COMMAND : Inport  Port=4
  ESTIMATED PITCH : Inport  Port=5
  ESTIMATED ROLL : Inport  Port=6
  ESTIMATED YAW : Inport  Port=7
  ESTIMATED ALTITUDE : Inport  Port=8
  ESTIMATED AIRSPEED : Inport  Port=9
  ALTITUDE COMMAND : Inport  Port=10
  " ALTITUDE ERROR" : Sum  Inputs=+-
  " PITCH ERROR" : Sum  Inputs=+-
  " ROLL ERROR" : Sum  Inputs=+-
  " SPEED ERROR" : Sum  Inputs=+-
  " YAW ERROR" : Sum  Inputs=+-
  AILERON LIMIT : Saturate  UpperLimit=1  LowerLimit=-1
  ALTITUDE PID : simulink/Continuous/PID Controller  Controller=PID  TimeDomain=Continuous-time  SampleTime=-1  IntegratorMethod=Forward Euler  FilterMethod=Forward Euler  Form=Parallel  UseFilter=on  ControllerParametersSource=internal  P=0.8  I=0.2  D=0  N=100  InitialConditionSource=internal  InitialConditionForIntegrator=0  InitialConditionForFilter=0  ExternalReset=none  LimitOutput=off  UpperSaturationLimit=inf  LowerSaturationLimit=-inf  LinearizeAsGain=on  AntiWindupMode=none  Kb=1  TrackingMode=off  Kt=1  PParamMin=[]  PParamMax=[]  IParamMin=[]  IParamMax=[]  DParamMin=[]  DParamMax=[]  NParamMin=[]  NParamMax=[]  KbParamMin=[]  KbParamMax=[]  KtParamMin=[]  KtParamMax=[]  POutMin=[]  POutMax=[]  IOutMin=[]  IOutMax=[]  DOutMin=[]  DOutMax=[]  NOutMin=[]  NOutMax=[]  KbOutMin=[]  KbOutMax=[]  KtOutMin=[]  KtOutMax=[]  IntegratorOutMin=[]  IntegratorOutMax=[]  FilterOutMin=[]  FilterOutMax=[]  SumOutMin=[]  SumOutMax=[]  SumI1OutMin=[]  SumI1OutMax=[]  SumI2OutMin=[]  SumI2OutMax=[]  SumI3OutMin=[]  SumI3OutMax=[]  SumDOutMin=[]  SumDOutMax=[]  SaturationOutMin=[]  SaturationOutMax=[]  IntegratorContinuousStateAttributes=''  IntegratorStateMustResolveToSignalObject=off  IntegratorRTWStateStorageClass=Auto  FilterContinuousStateAttributes=''  FilterStateMustResolveToSignalObject=off  FilterRTWStateStorageClass=Auto  DifferentiatorICPrevScaledInput=0  DifferentiatorOutMin=[]  DifferentiatorOutMax=[]  FilterDiffOutCoefMin=[]  FilterDiffOutCoefMax=[]  SumDenOutMin=[]  SumDenOutMax=[]  SumNumOutMin=[]  SumNumOutMax=[]  ReciprocalOutMin=[]  ReciprocalOutMax=[]  DivideOutMin=[]  DivideOutMax=[]  TunerSelectOption=Transfer Function Based (PID Tuner App)
  Constant : Constant  Value=0
  Display{,1..4} (5 alike) : Display
  ELEVATOR LIMIT : Saturate  UpperLimit=1  LowerLimit=-1
  PITCH MODE SELECT : Switch  Criteria=u2 > Threshold
  PITCH PID : simulink/Continuous/PID Controller  Controller=PID  TimeDomain=Continuous-time  SampleTime=-1  IntegratorMethod=Forward Euler  FilterMethod=Forward Euler  Form=Parallel  UseFilter=on  ControllerParametersSource=internal  P=2  I=0.5  D=0.1  N=100  InitialConditionSource=internal  InitialConditionForIntegrator=0  InitialConditionForFilter=0  ExternalReset=none  LimitOutput=off  UpperSaturationLimit=inf  LowerSaturationLimit=-inf  LinearizeAsGain=on  AntiWindupMode=none  Kb=1  TrackingMode=off  Kt=1  PParamMin=[]  PParamMax=[]  IParamMin=[]  IParamMax=[]  DParamMin=[]  DParamMax=[]  NParamMin=[]  NParamMax=[]  KbParamMin=[]  KbParamMax=[]  KtParamMin=[]  KtParamMax=[]  POutMin=[]  POutMax=[]  IOutMin=[]  IOutMax=[]  DOutMin=[]  DOutMax=[]  NOutMin=[]  NOutMax=[]  KbOutMin=[]  KbOutMax=[]  KtOutMin=[]  KtOutMax=[]  IntegratorOutMin=[]  IntegratorOutMax=[]  FilterOutMin=[]  FilterOutMax=[]  SumOutMin=[]  SumOutMax=[]  SumI1OutMin=[]  SumI1OutMax=[]  SumI2OutMin=[]  SumI2OutMax=[]  SumI3OutMin=[]  SumI3OutMax=[]  SumDOutMin=[]  SumDOutMax=[]  SaturationOutMin=[]  SaturationOutMax=[]  IntegratorContinuousStateAttributes=''  IntegratorStateMustResolveToSignalObject=off  IntegratorRTWStateStorageClass=Auto  FilterContinuousStateAttributes=''  FilterStateMustResolveToSignalObject=off  FilterRTWStateStorageClass=Auto  DifferentiatorICPrevScaledInput=0  DifferentiatorOutMin=[]  DifferentiatorOutMax=[]  FilterDiffOutCoefMin=[]  FilterDiffOutCoefMax=[]  SumDenOutMin=[]  SumDenOutMax=[]  SumNumOutMin=[]  SumNumOutMax=[]  ReciprocalOutMin=[]  ReciprocalOutMax=[]  DivideOutMin=[]  DivideOutMax=[]  TunerSelectOption=Transfer Function Based (PID Tuner App)
  ROLL PID : simulink/Continuous/PID Controller  Controller=PID  TimeDomain=Continuous-time  SampleTime=-1  IntegratorMethod=Forward Euler  FilterMethod=Forward Euler  Form=Parallel  UseFilter=on  ControllerParametersSource=internal  P=2  I=0.5  D=0.1  N=100  InitialConditionSource=internal  InitialConditionForIntegrator=0  InitialConditionForFilter=0  ExternalReset=none  LimitOutput=off  UpperSaturationLimit=inf  LowerSaturationLimit=-inf  LinearizeAsGain=on  AntiWindupMode=none  Kb=1  TrackingMode=off  Kt=1  PParamMin=[]  PParamMax=[]  IParamMin=[]  IParamMax=[]  DParamMin=[]  DParamMax=[]  NParamMin=[]  NParamMax=[]  KbParamMin=[]  KbParamMax=[]  KtParamMin=[]  KtParamMax=[]  POutMin=[]  POutMax=[]  IOutMin=[]  IOutMax=[]  DOutMin=[]  DOutMax=[]  NOutMin=[]  NOutMax=[]  KbOutMin=[]  KbOutMax=[]  KtOutMin=[]  KtOutMax=[]  IntegratorOutMin=[]  IntegratorOutMax=[]  FilterOutMin=[]  FilterOutMax=[]  SumOutMin=[]  SumOutMax=[]  SumI1OutMin=[]  SumI1OutMax=[]  SumI2OutMin=[]  SumI2OutMax=[]  SumI3OutMin=[]  SumI3OutMax=[]  SumDOutMin=[]  SumDOutMax=[]  SaturationOutMin=[]  SaturationOutMax=[]  IntegratorContinuousStateAttributes=''  IntegratorStateMustResolveToSignalObject=off  IntegratorRTWStateStorageClass=Auto  FilterContinuousStateAttributes=''  FilterStateMustResolveToSignalObject=off  FilterRTWStateStorageClass=Auto  DifferentiatorICPrevScaledInput=0  DifferentiatorOutMin=[]  DifferentiatorOutMax=[]  FilterDiffOutCoefMin=[]  FilterDiffOutCoefMax=[]  SumDenOutMin=[]  SumDenOutMax=[]  SumNumOutMin=[]  SumNumOutMax=[]  ReciprocalOutMin=[]  ReciprocalOutMax=[]  DivideOutMin=[]  DivideOutMax=[]  TunerSelectOption=Transfer Function Based (PID Tuner App)
  RUDDER LIMIT : Saturate  UpperLimit=1  LowerLimit=-1
  SPEED PID : simulink/Continuous/PID Controller  Controller=PID  TimeDomain=Continuous-time  SampleTime=-1  IntegratorMethod=Forward Euler  FilterMethod=Forward Euler  Form=Parallel  UseFilter=on  ControllerParametersSource=internal  P=2  I=0.5  D=0.1  N=100  InitialConditionSource=internal  InitialConditionForIntegrator=0  InitialConditionForFilter=0  ExternalReset=none  LimitOutput=off  UpperSaturationLimit=inf  LowerSaturationLimit=-inf  LinearizeAsGain=on  AntiWindupMode=none  Kb=1  TrackingMode=off  Kt=1  PParamMin=[]  PParamMax=[]  IParamMin=[]  IParamMax=[]  DParamMin=[]  DParamMax=[]  NParamMin=[]  NParamMax=[]  KbParamMin=[]  KbParamMax=[]  KtParamMin=[]  KtParamMax=[]  POutMin=[]  POutMax=[]  IOutMin=[]  IOutMax=[]  DOutMin=[]  DOutMax=[]  NOutMin=[]  NOutMax=[]  KbOutMin=[]  KbOutMax=[]  KtOutMin=[]  KtOutMax=[]  IntegratorOutMin=[]  IntegratorOutMax=[]  FilterOutMin=[]  FilterOutMax=[]  SumOutMin=[]  SumOutMax=[]  SumI1OutMin=[]  SumI1OutMax=[]  SumI2OutMin=[]  SumI2OutMax=[]  SumI3OutMin=[]  SumI3OutMax=[]  SumDOutMin=[]  SumDOutMax=[]  SaturationOutMin=[]  SaturationOutMax=[]  IntegratorContinuousStateAttributes=''  IntegratorStateMustResolveToSignalObject=off  IntegratorRTWStateStorageClass=Auto  FilterContinuousStateAttributes=''  FilterStateMustResolveToSignalObject=off  FilterRTWStateStorageClass=Auto  DifferentiatorICPrevScaledInput=0  DifferentiatorOutMin=[]  DifferentiatorOutMax=[]  FilterDiffOutCoefMin=[]  FilterDiffOutCoefMax=[]  SumDenOutMin=[]  SumDenOutMax=[]  SumNumOutMin=[]  SumNumOutMax=[]  ReciprocalOutMin=[]  ReciprocalOutMax=[]  DivideOutMin=[]  DivideOutMax=[]  TunerSelectOption=Transfer Function Based (PID Tuner App)
  THROTTLE LIMIT : Saturate  UpperLimit=1  LowerLimit=0
  YAW PID : simulink/Continuous/PID Controller  Controller=PID  TimeDomain=Continuous-time  SampleTime=-1  IntegratorMethod=Forward Euler  FilterMethod=Forward Euler  Form=Parallel  UseFilter=on  ControllerParametersSource=internal  P=2  I=0.5  D=0.1  N=100  InitialConditionSource=internal  InitialConditionForIntegrator=0  InitialConditionForFilter=0  ExternalReset=none  LimitOutput=off  UpperSaturationLimit=inf  LowerSaturationLimit=-inf  LinearizeAsGain=on  AntiWindupMode=none  Kb=1  TrackingMode=off  Kt=1  PParamMin=[]  PParamMax=[]  IParamMin=[]  IParamMax=[]  DParamMin=[]  DParamMax=[]  NParamMin=[]  NParamMax=[]  KbParamMin=[]  KbParamMax=[]  KtParamMin=[]  KtParamMax=[]  POutMin=[]  POutMax=[]  IOutMin=[]  IOutMax=[]  DOutMin=[]  DOutMax=[]  NOutMin=[]  NOutMax=[]  KbOutMin=[]  KbOutMax=[]  KtOutMin=[]  KtOutMax=[]  IntegratorOutMin=[]  IntegratorOutMax=[]  FilterOutMin=[]  FilterOutMax=[]  SumOutMin=[]  SumOutMax=[]  SumI1OutMin=[]  SumI1OutMax=[]  SumI2OutMin=[]  SumI2OutMax=[]  SumI3OutMin=[]  SumI3OutMax=[]  SumDOutMin=[]  SumDOutMax=[]  SaturationOutMin=[]  SaturationOutMax=[]  IntegratorContinuousStateAttributes=''  IntegratorStateMustResolveToSignalObject=off  IntegratorRTWStateStorageClass=Auto  FilterContinuousStateAttributes=''  FilterStateMustResolveToSignalObject=off  FilterRTWStateStorageClass=Auto  DifferentiatorICPrevScaledInput=0  DifferentiatorOutMin=[]  DifferentiatorOutMax=[]  FilterDiffOutCoefMin=[]  FilterDiffOutCoefMax=[]  SumDenOutMin=[]  SumDenOutMax=[]  SumNumOutMin=[]  SumNumOutMax=[]  ReciprocalOutMin=[]  ReciprocalOutMax=[]  DivideOutMin=[]  DivideOutMax=[]  TunerSelectOption=Transfer Function Based (PID Tuner App)
  ELEVATOR : Outport
  AILERON : Outport  Port=2
  RUDDER : Outport  Port=3
  THROTTLE : Outport  Port=4
  wires:
  ESTIMATED PITCH/1 -> " PITCH ERROR"/2
  AILERON COMMAND/1 -> " ROLL ERROR"/1
  ESTIMATED ROLL/1 -> " ROLL ERROR"/2
  RUDDER COMMAND/1 -> " YAW ERROR"/1
  ESTIMATED YAW/1 -> " YAW ERROR"/2
  THROTTLE COMMAND/1 -> " SPEED ERROR"/1
  ESTIMATED AIRSPEED/1 -> " SPEED ERROR"/2
  " PITCH ERROR"/1 -> PITCH PID/1, Display/1
  " ROLL ERROR"/1 -> ROLL PID/1, Display1/1
  " YAW ERROR"/1 -> YAW PID/1, Display2/1
  " SPEED ERROR"/1 -> SPEED PID/1, Display3/1
  PITCH PID/1 -> ELEVATOR LIMIT/1
  ELEVATOR LIMIT/1 -> ELEVATOR/1
  ROLL PID/1 -> AILERON LIMIT/1
  AILERON LIMIT/1 -> AILERON/1
  YAW PID/1 -> RUDDER LIMIT/1
  RUDDER LIMIT/1 -> RUDDER/1
  SPEED PID/1 -> THROTTLE LIMIT/1
  THROTTLE LIMIT/1 -> THROTTLE/1
  ALTITUDE COMMAND/1 -> " ALTITUDE ERROR"/1
  ESTIMATED ALTITUDE/1 -> " ALTITUDE ERROR"/2
  " ALTITUDE ERROR"/1 -> ALTITUDE PID/1, Display4/1
  PITCH COMMAND/1 -> PITCH MODE SELECT/1
  ALTITUDE PID/1 -> PITCH MODE SELECT/3
  Constant/1 -> PITCH MODE SELECT/2
  PITCH MODE SELECT/1 -> " PITCH ERROR"/1

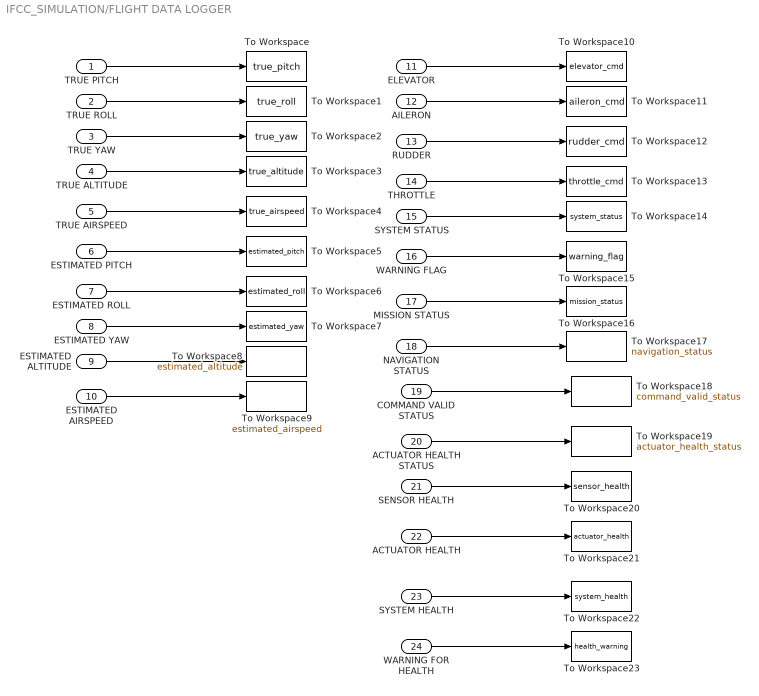
== system IFCC_SIMULATION/FLIGHT DATA LOGGER ==
  TRUE PITCH : Inport
  TRUE ROLL : Inport  Port=2
  TRUE YAW : Inport  Port=3
  TRUE ALTITUDE : Inport  Port=4
  TRUE AIRSPEED : Inport  Port=5
  ESTIMATED PITCH : Inport  Port=6
  ESTIMATED ROLL : Inport  Port=7
  ESTIMATED YAW : Inport  Port=8
  ESTIMATED ALTITUDE : Inport  Port=9
  ESTIMATED AIRSPEED : Inport  Port=10
  ELEVATOR : Inport  Port=11
  AILERON : Inport  Port=12
  RUDDER : Inport  Port=13
  THROTTLE : Inport  Port=14
  SYSTEM STATUS : Inport  Port=15
  WARNING FLAG : Inport  Port=16
  MISSION STATUS : Inport  Port=17
  NAVIGATION STATUS : Inport  Port=18
  COMMAND VALID STATUS : Inport  Port=19
  ACTUATOR HEALTH STATUS : Inport  Port=20
  SENSOR HEALTH : Inport  Port=21
  ACTUATOR HEALTH : Inport  Port=22
  SYSTEM HEALTH : Inport  Port=23
  WARNING FOR HEALTH : Inport  Port=24
  To Workspace : ToWorkspace  VariableName=true_pitch  SampleTime=-1
  To Workspace1 : ToWorkspace  VariableName=true_roll  SampleTime=-1
  To Workspace10 : ToWorkspace  VariableName=elevator_cmd  SampleTime=-1
  To Workspace11 : ToWorkspace  VariableName=aileron_cmd  SampleTime=-1
  To Workspace12 : ToWorkspace  VariableName=rudder_cmd  SampleTime=-1
  To Workspace13 : ToWorkspace  VariableName=throttle_cmd  SampleTime=-1
  To Workspace14 : ToWorkspace  VariableName=system_status  SampleTime=-1
  To Workspace15 : ToWorkspace  VariableName=warning_flag  SampleTime=-1
  To Workspace16 : ToWorkspace  VariableName=mission_status  SampleTime=-1
  To Workspace17 : ToWorkspace  VariableName=navigation_status  SampleTime=-1
  To Workspace18 : ToWorkspace  VariableName=command_valid_status  SampleTime=-1
  To Workspace19 : ToWorkspace  VariableName=actuator_health_status  SampleTime=-1
  To Workspace2 : ToWorkspace  VariableName=true_yaw  SampleTime=-1
  To Workspace20 : ToWorkspace  VariableName=sensor_health  SampleTime=-1
  To Workspace21 : ToWorkspace  VariableName=actuator_health  SampleTime=-1
  To Workspace22 : ToWorkspace  VariableName=system_health  SampleTime=-1
  To Workspace23 : ToWorkspace  VariableName=health_warning  SampleTime=-1
  To Workspace3 : ToWorkspace  VariableName=true_altitude  SampleTime=-1
  To Workspace4 : ToWorkspace  VariableName=true_airspeed  SampleTime=-1
  To Workspace5 : ToWorkspace  VariableName=estimated_pitch  SampleTime=-1
  To Workspace6 : ToWorkspace  VariableName=estimated_roll  SampleTime=-1
  To Workspace7 : ToWorkspace  VariableName=estimated_yaw  SampleTime=-1
  To Workspace8 : ToWorkspace  VariableName=estimated_altitude  SampleTime=-1
  To Workspace9 : ToWorkspace  VariableName=estimated_airspeed  SampleTime=-1
  wires:
  TRUE PITCH/1 -> To Workspace/1
  TRUE ROLL/1 -> To Workspace1/1
  TRUE YAW/1 -> To Workspace2/1
  TRUE ALTITUDE/1 -> To Workspace3/1
  TRUE AIRSPEED/1 -> To Workspace4/1
  ESTIMATED PITCH/1 -> To Workspace5/1
  ESTIMATED ROLL/1 -> To Workspace6/1
  ESTIMATED YAW/1 -> To Workspace7/1
  ESTIMATED ALTITUDE/1 -> To Workspace8/1
  ESTIMATED AIRSPEED/1 -> To Workspace9/1
  ELEVATOR/1 -> To Workspace10/1
  AILERON/1 -> To Workspace11/1
  RUDDER/1 -> To Workspace12/1
  THROTTLE/1 -> To Workspace13/1
  SYSTEM STATUS/1 -> To Workspace14/1
  WARNING FLAG/1 -> To Workspace15/1
  MISSION STATUS/1 -> To Workspace16/1
  NAVIGATION STATUS/1 -> To Workspace17/1
  COMMAND VALID STATUS/1 -> To Workspace18/1
  ACTUATOR HEALTH STATUS/1 -> To Workspace19/1
  SENSOR HEALTH/1 -> To Workspace20/1
  ACTUATOR HEALTH/1 -> To Workspace21/1
  SYSTEM HEALTH/1 -> To Workspace22/1
  WARNING FOR HEALTH/1 -> To Workspace23/1

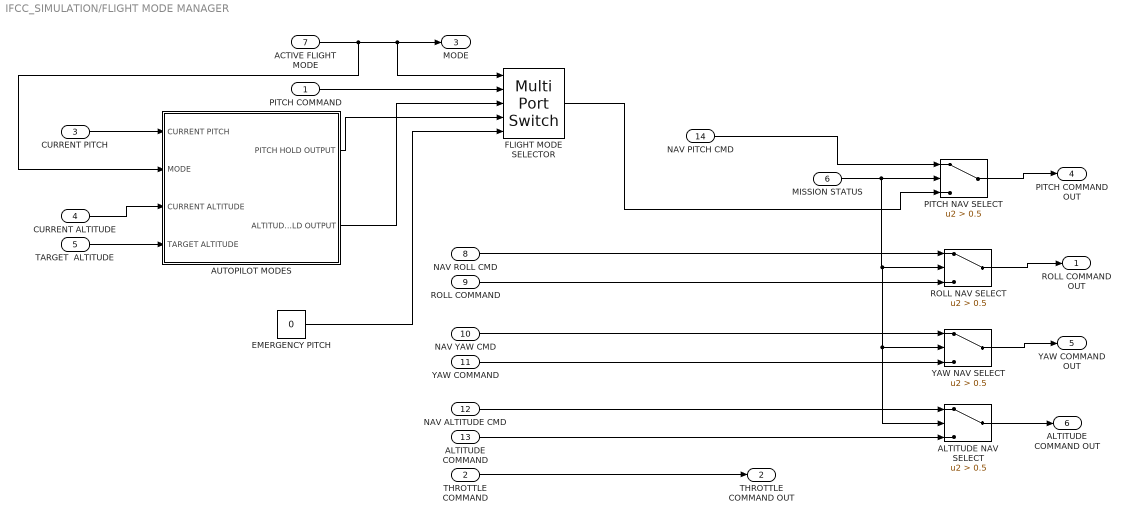
== system IFCC_SIMULATION/FLIGHT MODE MANAGER ==
  PITCH COMMAND : Inport
  THROTTLE COMMAND : Inport  Port=2
  CURRENT PITCH : Inport  Port=3
  CURRENT ALTITUDE : Inport  Port=4
  TARGET  ALTITUDE : Inport  Port=5
  MISSION STATUS : Inport  Port=6
  ACTIVE FLIGHT MODE : Inport  Port=7
  NAV ROLL CMD : Inport  Port=8
  ROLL COMMAND : Inport  Port=9
  NAV YAW CMD : Inport  Port=10
  YAW COMMAND : Inport  Port=11
  NAV ALTITUDE CMD : Inport  Port=12
  ALTITUDE COMMAND : Inport  Port=13
  NAV PITCH CMD : Inport  Port=14
  ALTITUDE NAV SELECT : Switch  Criteria=u2 > Threshold  Threshold=0.5
  AUTOPILOT MODES : Subsystem
  EMERGENCY PITCH : Constant  Value=0
  "FLIGHT MODE SELECTOR " : MultiPortSwitch  Inputs=4
  PITCH NAV SELECT : Switch  Criteria=u2 > Threshold  Threshold=0.5
  ROLL NAV SELECT : Switch  Criteria=u2 > Threshold  Threshold=0.5
  YAW NAV SELECT : Switch  Criteria=u2 > Threshold  Threshold=0.5
  ROLL COMMAND OUT : Outport
  THROTTLE COMMAND OUT : Outport  Port=2
  MODE : Outport  Port=3
  "PITCH COMMAND OUT " : Outport  Port=4
  YAW COMMAND OUT : Outport  Port=5
  ALTITUDE COMMAND OUT : Outport  Port=6
  wires:
  NAV YAW CMD/1 -> YAW NAV SELECT/1
  THROTTLE COMMAND/1 -> THROTTLE COMMAND OUT/1
  PITCH COMMAND/1 -> "FLIGHT MODE SELECTOR "/2
  NAV ALTITUDE CMD/1 -> ALTITUDE NAV SELECT/1
  ACTIVE FLIGHT MODE/1 -> MODE/1, "FLIGHT MODE SELECTOR "/1, AUTOPILOT MODES/2(MODE)
  EMERGENCY PITCH/1 -> "FLIGHT MODE SELECTOR "/5
  AUTOPILOT MODES/1(PITCH HOLD OUTPUT) -> "FLIGHT MODE SELECTOR "/4
  AUTOPILOT MODES/2(ALTITUDE HOLD OUTPUT) -> "FLIGHT MODE SELECTOR "/3
  CURRENT PITCH/1 -> AUTOPILOT MODES/1(CURRENT PITCH)
  CURRENT ALTITUDE/1 -> AUTOPILOT MODES/3(CURRENT ALTITUDE)
  TARGET  ALTITUDE/1 -> AUTOPILOT MODES/4(TARGET ALTITUDE)
  "FLIGHT MODE SELECTOR "/1 -> PITCH NAV SELECT/3
  MISSION STATUS/1 -> ALTITUDE NAV SELECT/2, YAW NAV SELECT/2, ROLL NAV SELECT/2, PITCH NAV SELECT/2
  PITCH NAV SELECT/1 -> "PITCH COMMAND OUT "/1
  ROLL NAV SELECT/1 -> ROLL COMMAND OUT/1
  NAV ROLL CMD/1 -> ROLL NAV SELECT/1
  ROLL COMMAND/1 -> ROLL NAV SELECT/3
  YAW NAV SELECT/1 -> YAW COMMAND OUT/1
  YAW COMMAND/1 -> YAW NAV SELECT/3
  ALTITUDE COMMAND/1 -> ALTITUDE NAV SELECT/3
  ALTITUDE NAV SELECT/1 -> ALTITUDE COMMAND OUT/1
  NAV PITCH CMD/1 -> PITCH NAV SELECT/1

== system IFCC_SIMULATION/HEALTH MONITORING ==
  IMU FAULT : Inport
  GPS FAULT : Inport  Port=2
  PITOT FAULT : Inport  Port=3
  ACTUATOR FAULT STATUS : Inport  Port=4
  COMMAND VALID STATUS : Inport  Port=5
  NAVIGATION STATUS : Inport  Port=6
  " LOGIC" : Logic  Operator=NOT  Inputs=3  AllPortsSameDT=off  OutDataTypeStr=boolean
  ACTUATOR HEALTH LOGIC : Logic  Operator=NOT  Inputs=3  AllPortsSameDT=off  OutDataTypeStr=boolean
  SENSOR FAULT AGGREGATOR : Logic  Operator=OR  Inputs=3  AllPortsSameDT=off  OutDataTypeStr=boolean
  SENSOR HEALTH LOGIC : Logic  Operator=NOT  Inputs=3  AllPortsSameDT=off  OutDataTypeStr=boolean
  SYSTEM HEALTH LOGIC : Logic  Inputs=3  AllPortsSameDT=off  OutDataTypeStr=boolean
  SYSTEM WARNING LOGIC : Logic  Operator=OR  Inputs=5  AllPortsSameDT=off  OutDataTypeStr=boolean
  SENSOR HEALTH : Outport
  ACTUATOR HEALTH : Outport  Port=2
  SYSTEM HEALTH : Outport  Port=3
  WARNING FLAG : Outport  Port=4
  wires:
  IMU FAULT/1 -> SYSTEM WARNING LOGIC/1, SENSOR FAULT AGGREGATOR/1
  GPS FAULT/1 -> SYSTEM WARNING LOGIC/2, SENSOR FAULT AGGREGATOR/2
  PITOT FAULT/1 -> SYSTEM WARNING LOGIC/3, SENSOR FAULT AGGREGATOR/3
  SENSOR FAULT AGGREGATOR/1 -> SENSOR HEALTH LOGIC/1
  SENSOR HEALTH LOGIC/1 -> SYSTEM HEALTH LOGIC/1, SENSOR HEALTH/1
  ACTUATOR FAULT STATUS/1 -> SYSTEM WARNING LOGIC/4, ACTUATOR HEALTH LOGIC/1
  ACTUATOR HEALTH LOGIC/1 -> SYSTEM HEALTH LOGIC/2, ACTUATOR HEALTH/1
  COMMAND VALID STATUS/1 -> SYSTEM HEALTH LOGIC/3, " LOGIC"/1
  SYSTEM WARNING LOGIC/1 -> WARNING FLAG/1
  SYSTEM HEALTH LOGIC/1 -> SYSTEM HEALTH/1
  " LOGIC"/1 -> SYSTEM WARNING LOGIC/5

== system IFCC_SIMULATION/NAVIGATION MANAGER ==
  ESTIMATED PITCH : Inport
  ESTIMATED ROLL : Inport  Port=2
  ESTIMATED YAW : Inport  Port=3
  ESTIMATED ALTITUDE : Inport  Port=4
  ESTIMATED AIRSPEED : Inport  Port=5
  TARGET WAYPOINT : Inport  Port=6
  MISSION STATUS : Inport  Port=7
  " YAW ERROR" : Sum  Inputs=+-
  ALTITUDE ERROR : Sum  Inputs=+-
  NAV PITCH LIMIT : Saturate  UpperLimit=0.3  LowerLimit=-0.3
  NAV ROLL REFERENCE : Constant  Value=0
  NAV YAW LIMIT : Saturate  UpperLimit=0.3  LowerLimit=-0.3
  PITCH GUIDANCE GAIN : Gain  Gain=0.01
  TARGET ALTITUDE : Constant  Value=100
  YAW GUIDANCE GAIN : Gain  Gain=0.01
  NAV PITCH CMD : Outport
  NAV ROLL CMD : Outport  Port=2
  NAV YAW CMD : Outport  Port=3
  NAV ALTITUDE CMD : Outport  Port=4
  NAVIGATION STATUS : Outport  Port=5
  wires:
  TARGET ALTITUDE/1 -> NAV ALTITUDE CMD/1, ALTITUDE ERROR/1
  ESTIMATED ALTITUDE/1 -> ALTITUDE ERROR/2
  ALTITUDE ERROR/1 -> PITCH GUIDANCE GAIN/1
  PITCH GUIDANCE GAIN/1 -> NAV PITCH LIMIT/1
  NAV PITCH LIMIT/1 -> NAV PITCH CMD/1
  NAV ROLL REFERENCE/1 -> NAV ROLL CMD/1
  TARGET WAYPOINT/1 -> " YAW ERROR"/1
  ESTIMATED YAW/1 -> " YAW ERROR"/2
  " YAW ERROR"/1 -> YAW GUIDANCE GAIN/1
  YAW GUIDANCE GAIN/1 -> NAV YAW LIMIT/1
  NAV YAW LIMIT/1 -> NAV YAW CMD/1
  MISSION STATUS/1 -> NAVIGATION STATUS/1

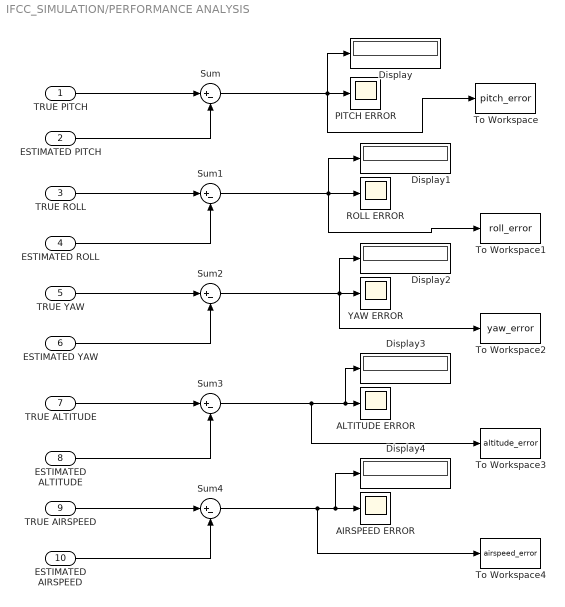
== system IFCC_SIMULATION/PERFORMANCE ANALYSIS ==
  TRUE PITCH : Inport
  ESTIMATED PITCH : Inport  Port=2
  TRUE ROLL : Inport  Port=3
  ESTIMATED ROLL : Inport  Port=4
  TRUE YAW : Inport  Port=5
  ESTIMATED YAW : Inport  Port=6
  TRUE ALTITUDE : Inport  Port=7
  ESTIMATED ALTITUDE : Inport  Port=8
  TRUE AIRSPEED : Inport  Port=9
  ESTIMATED AIRSPEED : Inport  Port=10
  AIRSPEED ERROR : Scope
  ALTITUDE ERROR : Scope
  Display{,1..4} (5 alike) : Display
  PITCH ERROR : Scope
  ROLL ERROR : Scope
  Sum{,1..4} (5 alike) : Sum  Inputs=|+-
  To Workspace : ToWorkspace  VariableName=pitch_error  SampleTime=-1
  To Workspace1 : ToWorkspace  VariableName=roll_error  SampleTime=-1
  To Workspace2 : ToWorkspace  VariableName=yaw_error  SampleTime=-1
  To Workspace3 : ToWorkspace  VariableName=altitude_error  SampleTime=-1
  To Workspace4 : ToWorkspace  VariableName=airspeed_error  SampleTime=-1
  YAW ERROR : Scope
  wires:
  TRUE PITCH/1 -> Sum/1
  ESTIMATED PITCH/1 -> Sum/2
  TRUE ROLL/1 -> Sum1/1
  ESTIMATED ROLL/1 -> Sum1/2
  TRUE YAW/1 -> Sum2/1
  ESTIMATED YAW/1 -> Sum2/2
  TRUE ALTITUDE/1 -> Sum3/1
  ESTIMATED ALTITUDE/1 -> Sum3/2
  TRUE AIRSPEED/1 -> Sum4/1
  ESTIMATED AIRSPEED/1 -> Sum4/2
  Sum/1 -> To Workspace/1, Display/1, PITCH ERROR/1
  Sum1/1 -> To Workspace1/1, Display1/1, ROLL ERROR/1
  Sum2/1 -> To Workspace2/1, Display2/1, YAW ERROR/1
  Sum3/1 -> To Workspace3/1, Display3/1, ALTITUDE ERROR/1
  Sum4/1 -> To Workspace4/1, Display4/1, AIRSPEED ERROR/1

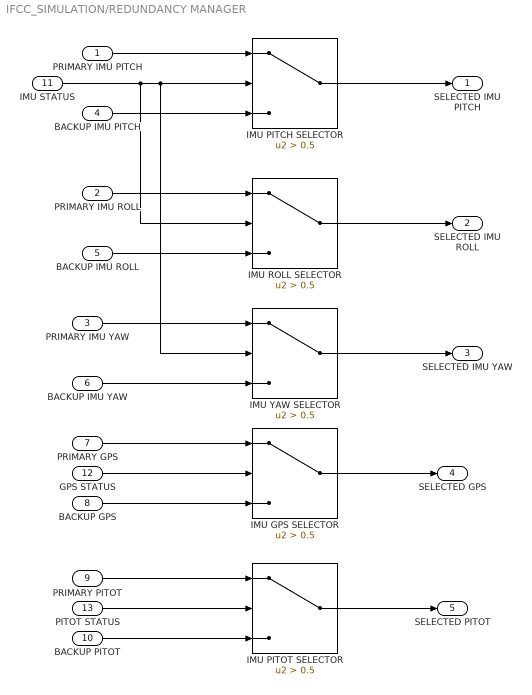
== system IFCC_SIMULATION/REDUNDANCY MANAGER ==
  PRIMARY IMU PITCH : Inport
  PRIMARY IMU ROLL : Inport  Port=2
  PRIMARY IMU YAW : Inport  Port=3
  BACKUP IMU PITCH : Inport  Port=4
  BACKUP IMU ROLL : Inport  Port=5
  BACKUP IMU YAW : Inport  Port=6
  PRIMARY GPS : Inport  Port=7
  BACKUP GPS : Inport  Port=8
  PRIMARY PITOT : Inport  Port=9
  BACKUP PITOT : Inport  Port=10
  IMU STATUS : Inport  Port=11
  GPS STATUS : Inport  Port=12
  PITOT STATUS : Inport  Port=13
  IMU GPS SELECTOR : Switch  Criteria=u2 > Threshold  Threshold=0.5
  IMU PITCH SELECTOR : Switch  Criteria=u2 > Threshold  Threshold=0.5
  IMU PITOT SELECTOR : Switch  Criteria=u2 > Threshold  Threshold=0.5
  IMU ROLL SELECTOR : Switch  Criteria=u2 > Threshold  Threshold=0.5
  IMU YAW SELECTOR : Switch  Criteria=u2 > Threshold  Threshold=0.5
  SELECTED IMU PITCH : Outport
  SELECTED IMU ROLL : Outport  Port=2
  SELECTED IMU YAW : Outport  Port=3
  SELECTED GPS : Outport  Port=4
  SELECTED PITOT : Outport  Port=5
  wires:
  PRIMARY IMU PITCH/1 -> IMU PITCH SELECTOR/1
  IMU STATUS/1 -> IMU ROLL SELECTOR/2, IMU YAW SELECTOR/2, IMU PITCH SELECTOR/2
  BACKUP IMU PITCH/1 -> IMU PITCH SELECTOR/3
  IMU PITCH SELECTOR/1 -> SELECTED IMU PITCH/1
  PRIMARY IMU ROLL/1 -> IMU ROLL SELECTOR/1
  BACKUP IMU ROLL/1 -> IMU ROLL SELECTOR/3
  IMU ROLL SELECTOR/1 -> SELECTED IMU ROLL/1
  PRIMARY IMU YAW/1 -> IMU YAW SELECTOR/1
  BACKUP IMU YAW/1 -> IMU YAW SELECTOR/3
  PRIMARY GPS/1 -> IMU GPS SELECTOR/1
  BACKUP GPS/1 -> IMU GPS SELECTOR/3
  IMU YAW SELECTOR/1 -> SELECTED IMU YAW/1
  IMU GPS SELECTOR/1 -> SELECTED GPS/1
  PRIMARY PITOT/1 -> IMU PITOT SELECTOR/1
  BACKUP PITOT/1 -> IMU PITOT SELECTOR/3
  IMU PITOT SELECTOR/1 -> SELECTED PITOT/1
  GPS STATUS/1 -> IMU GPS SELECTOR/2
  PITOT STATUS/1 -> IMU PITOT SELECTOR/2

== system IFCC_SIMULATION/SENSOR SIMULATION ==
  Pitch : Inport
  Roll : Inport  Port=2
  Yaw : Inport  Port=3
  Altitude : Inport  Port=4
  Airspeed : Inport  Port=5
  " GPS Sensor" : Subsystem
  " IMU Pitch Sensor " : Subsystem
  " IMU Roll Sensor" : Subsystem
  " IMU Yaw Sensor" : Subsystem
  PITOT AIRSPEED SENSOR : Subsystem
  IMU Pitch : Outport
  IMU Roll : Outport  Port=2
  IMU Yaw : Outport  Port=3
  GPS Altitude : Outport  Port=4
  Pitot Airspeed : Outport  Port=5
  wires:
  Pitch/1 -> " IMU Pitch Sensor "/1(TRUE ANGLE)
  " IMU Pitch Sensor "/1(MEASURED ANGLE) -> IMU Pitch/1
  Roll/1 -> " IMU Roll Sensor"/1(TRUE ANGLE)
  Yaw/1 -> " IMU Yaw Sensor"/1(TRUE ANGLE)
  " IMU Roll Sensor"/1(MEASURED ANGLE) -> IMU Roll/1
  " IMU Yaw Sensor"/1(MEASURED ANGLE) -> IMU Yaw/1
  Altitude/1 -> " GPS Sensor"/1(TRUE ALTITUDE)
  " GPS Sensor"/1(GPS ALTITUDE) -> GPS Altitude/1
  Airspeed/1 -> PITOT AIRSPEED SENSOR/1(TRUE AIRSPEED)
  PITOT AIRSPEED SENSOR/1(PITOT AIRSPEED) -> Pitot Airspeed/1
